simulink model "Auto_Coffee"  (R2017a)
settings: Solver=VariableStepAuto  StartTime=0.0  StopTime=25  RelTol=1e-3
undefined symbols (not defined in the file): sigbuilder_block
settings Model: Creator=Administrator  LastModifiedBy=Administrator
settings OptimizationCC: DefaultParameterBehavior=Inlined  UseDivisionForNetSlopeComputation=on  UseFloatMulNetSlope=on  InlineInvariantSignals=on  PassReuseOutputArgsAs=Individual arguments  ZeroExternalMemoryAtStartup=off  ZeroInternalMemoryAtStartup=off  NoFixptDivByZeroProtection=on  EfficientFloat2IntCast=on  LifeSpan=1
settings DebuggingCC: ParameterTunabilityLossMsg=error
settings HardwareCC: ProdBitPerPointer=32  ProdBitPerSizeT=32  ProdBitPerPtrDiffT=32  ProdLargestAtomicInteger=Long  ProdWordSize=32  ProdHWDeviceType=ARM Compatible->ARM 7
settings SFSimCC: MATLABDynamicMemAlloc=off
settings RTWCC: SystemTargetFile=ert.tlc  TemplateMakefile=ert_default_tmf  Description=Embedded Coder  GenerateReport=on  IncludeHyperlinkInReport=on  LaunchReport=on  GenerateTraceInfo=on  GenerateTraceReport=on  GenerateTraceReportSl=on  GenerateTraceReportSf=on  GenerateTraceReportEml=on  GenerateCodeMetricsReport=on
settings CodeAppCC: ForceParamTrailComments=on  IgnoreCustomStorageClasses=off  OperatorAnnotations=on  SimulinkDataObjDesc=on  SFDataObjDesc=on  MATLABFcnDesc=on  CustomSymbolStrGlobalVar=rt$N$M  CustomSymbolStrType=$N$M  CustomSymbolStrFcn=$N$M$F  CustomSymbolStrMacro=$N$M  InsertBlockDesc=on  MATLABSourceComments=on
settings ERTTargetCC: TargetLangStandard=C99 (ISO)  GenerateSampleERTMain=on  IncludeMdlTerminateFcn=off  CombineSignalStateStructs=on  SupportComplex=off  SupportContinuousTime=on  SupportNonInlinedSFcns=on  InlinedParameterPlacement=NonHierarchical  ERTCustomFileTemplate=example_file_process.tlc  ERTFilePackagingFormat=CompactWithDataFile

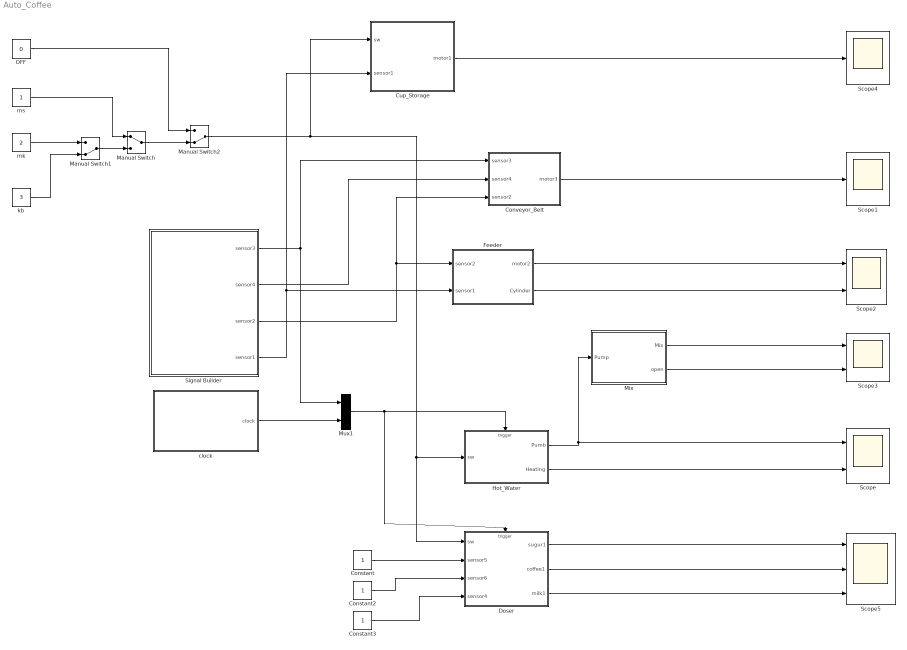
== system Auto_Coffee ==
  Constant : Constant
  Constant2 : Constant
  Constant3 : Constant
  Conveyor_Belt : Stateflow chart  TreatAsAtomicUnit=on
  Cup_Storage : Stateflow chart  TreatAsAtomicUnit=on
  Doser : Stateflow chart  TreatAsAtomicUnit=on
  Feeder : Stateflow chart  TreatAsAtomicUnit=on
  Hot_Water : Stateflow chart  TreatAsAtomicUnit=on
  Manual Switch : ManualSwitch
  Manual Switch1 : ManualSwitch  CurrentSetting=0
  Manual Switch2 : ManualSwitch  CurrentSetting=0
  Mix : Stateflow chart  TreatAsAtomicUnit=on
  Mux1 : Mux  Inputs=2
  OFF : Constant  Value=0
  Scope : Scope  NumInputPorts=2
  Scope1 : Scope
  Scope2 : Scope  NumInputPorts=2
  Scope3 : Scope  NumInputPorts=2
  Scope4 : Scope
  Scope5 : Scope  NumInputPorts=3
  Signal Builder : Subsystem  Tag=STV Subsys  LoadFcn=sigbuilder_block('load');  StartFcn=sigbuilder_block('start');  StopFcn=sigbuilder_block('stop');  ClipboardFcn=sigbuilder_block('clipboard');  mask(Sigbuilder block){tuvar=[0:10]}
      mask help: Simulink:masks:SigbuilderBlock_MD
      mask init:
      | if ~strcmp(get_param(bdroot(gcbh),'SimulationStatus'),'stopped') tuvar = sigbuilder_block('maskInit'); end
      settings: CopyFcn=sigbuilder_block('copy');  DeleteFcn=sigbuilder_block('delete');  ModelCloseFcn=sigbuilder_block('modelClose');  PreSaveFcn=sigbuilder_block('preSave');  PauseFcn=sigbuilder_block('pause');  ContinueFcn=sigbuilder_block('continue');  NameChangeFcn=sigbuilder_block('namechange');  OpenFcn=sigbuilder_block('open',[-90.75 166.5 572.25 408.75 ]);  CloseFcn=sigbuilder_block('close');
      mask Display: plot(0, 0, 100, 100,[2, 2, 32, 32, 2], [68, 8, 8, 68, 68],[32, 2], [38, 38], [32, 19, 2],[53, 60, 44], [32, 17, 17, 2],[16, 16, 31, 31]);txt = getActiveGroup(gcbh);text(2, 100, txt,'verticalAlignment', 'top');
  clock : Subsystem  Tag=STV Subsys  LoadFcn=sigbuilder_block('load');  StartFcn=sigbuilder_block('start');  StopFcn=sigbuilder_block('stop');  ClipboardFcn=sigbuilder_block('clipboard');  mask(Sigbuilder block){tuvar=[0:10]}
      mask help: Simulink:masks:SigbuilderBlock_MD
      mask init:
      | if ~strcmp(get_param(bdroot(gcbh),'SimulationStatus'),'stopped') tuvar = sigbuilder_block('maskInit'); end
      settings: CopyFcn=sigbuilder_block('copy');  DeleteFcn=sigbuilder_block('delete');  ModelCloseFcn=sigbuilder_block('modelClose');  PreSaveFcn=sigbuilder_block('preSave');  PauseFcn=sigbuilder_block('pause');  ContinueFcn=sigbuilder_block('continue');  NameChangeFcn=sigbuilder_block('namechange');  OpenFcn=sigbuilder_block('open',[517.5 155.25 550.5 358.5 ]);  CloseFcn=sigbuilder_block('close');
      mask Display: plot(0, 0, 100, 100,[2, 2, 32, 32, 2], [68, 8, 8, 68, 68],[32, 2], [38, 38], [32, 19, 2],[53, 60, 44], [32, 17, 17, 2],[16, 16, 31, 31]);txt = getActiveGroup(gcbh);text(2, 100, txt,'verticalAlignment', 'top');
  kb : Constant  Value=3
  mk : Constant  Value=2
  ms : Constant
  wires:
  Hot_Water/1(Pumb) -> Mix/1(Pump), Scope/1
  Hot_Water/2(Heating) -> Scope/2
  Signal Builder/1(sensor3) -> Conveyor_Belt/1(sensor3), Mux1/1
  Conveyor_Belt/1(motor3) -> Scope1/1
  Signal Builder/2(sensor4) -> Conveyor_Belt/2(sensor4)
  Signal Builder/3(sensor2) -> Conveyor_Belt/3(sensor2), Feeder/1(sensor2)
  Signal Builder/4(sensor1) -> Cup_Storage/2(sensor1), Feeder/2(sensor1)
  Feeder/1(motor2) -> Scope2/1
  Mix/1(Mix) -> Scope3/1
  Mix/2(open) -> Scope3/2
  Feeder/2(Cylinder) -> Scope2/2
  Cup_Storage/1(motor1) -> Scope4/1
  Constant/1 -> Doser/2(sensor5)
  Constant3/1 -> Doser/4(sensor4)
  Constant2/1 -> Doser/3(sensor6)
  clock/1(clock) -> Mux1/2
  Mux1/1 -> Hot_Water/Trigger, Doser/Trigger
  Manual Switch2/1 -> Hot_Water/1(sw), Doser/1(sw), Cup_Storage/1(sw)
  Manual Switch/1 -> Manual Switch2/2
  Manual Switch1/1 -> Manual Switch/2
  OFF/1 -> Manual Switch2/1
  ms/1 -> Manual Switch/1
  mk/1 -> Manual Switch1/1
  kb/1 -> Manual Switch1/2
  Doser/1(sugur1) -> Scope5/1
  Doser/2(coffee1) -> Scope5/2
  Doser/3(milk1) -> Scope5/3

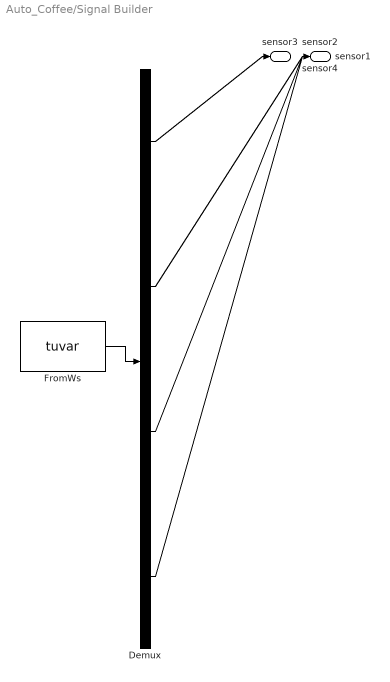
== system Auto_Coffee/Signal Builder ==
  Demux : Demux  Tag=STV Demux
  FromWs : FromWorkspace  Tag=STV FromWs  VariableName=tuvar  SampleTime=0
      SigBuilderData=|
      | common.afterFinalStr = 'Extrapolate'
      | common.sampleTime = 0
      | dataSet.timeRange = [0 25]
      | dataSet.name = 'Group 1'
      | sbobj.Groups.Name = 'Group 1'
      | sbobj.Groups.Signals(1).Name = 'sensor3'
      | sbobj.Groups.Signals(1).XData = [0 10 10 20 20 25]
      | sbobj.Groups.Signals(1).YData = [0 0 1 1 0 0]
      | sbobj.Groups.Signals(2).Name = 'sensor4'
      | sbobj.Groups.Signals(2).XData = [0 23 23 25]
      | sbobj.Groups.Signals(2).YData = [0 0 1 1]
      | sbobj.Groups.Signals(3).Name = 'sensor2'
      | sbobj.Groups.Signals(3).XData = [0 4 4 6 6 25]
      | sbobj.Groups.Signals(3).YData = [0 0 1 1 0 0]
      | sbobj.Groups.Signals(4).Name = 'sensor1'
      | sbobj.Groups.Signals(4).XData = [0 2 2 3 3 25]
      | sbobj.Groups.Signals(4).YData = [0 0 1 1 0 0]
      | sbobj.Groups.TimeRange = [0 25]
  sensor3 : Outport  Tag=STV Outport
  sensor4 : Outport  Tag=STV Outport  Port=2
  sensor2 : Outport  Tag=STV Outport  Port=3
  sensor1 : Outport  Tag=STV Outport  Port=4
  wires:
  FromWs/1 -> Demux/1
  Demux/1 -> sensor3/1
  Demux/2 -> sensor4/1
  Demux/3 -> sensor2/1
  Demux/4 -> sensor1/1

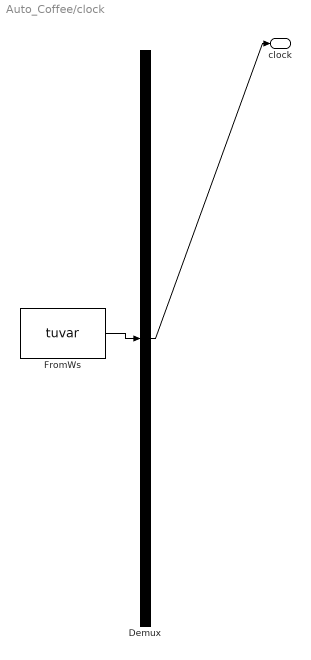
== system Auto_Coffee/clock ==
  Demux : Demux  Tag=STV Demux  Outputs=1
  FromWs : FromWorkspace  Tag=STV FromWs  VariableName=tuvar  SampleTime=0
      SigBuilderData=|
      | common.afterFinalStr = 'Extrapolate'
      | common.sampleTime = 0
      | dataSet.timeRange = [0 25]
      | dataSet.name = 'Group 1'
      | sbobj.Groups.Name = 'Group 1'
      | sbobj.Groups.Signals.Name = 'clock'
      | sbobj.Groups.Signals.XData = [0 0.25 0.25 0.5 0.5 0.75 0.75 1 1 1.25 1.25 1.5 1.5 1.75 1.75 2 2 2.25 2.25 2.5 2.5 2.75 2.75 3 3 3.25 3.25 3.5 3.5 3.75 3.75 4 4 4.25 4.25 4.5 4.5 4.75 4.75 5 5 5.25 5.25 5.5 5.5 5.75 5.75 6 6 6.25 6.25 6.5 6.5 6.75 6.75 7 7 7.25 7.25 7.5 7.5 7.75 7.75 8 8 8.25 8.25 8.5 8.5 8.75 8.75 9 9 9.25 9.25 9.5 9.5 9.75 9.75 10 10 10.25 10.25 10.5 10.5 10.75 10.75 11 11 11.25 11.25 11.5 11.5 11.75 11.75 12 12 12.25 12.25 12.5 12.5 12.75 12.75 13 13 13.25 13.25 13.5 13.5 13.75 13.75 14 14 14.25 14.25 14.5 14.5 14.75 14.75 15 15 15.25 15.25 15.5 15.5 15.75 15.75 16 16 16.25 16.25 16.5 16.5 16.75 16.75 17 17 17.25 17.25 17.5 17.5 17.75 17.75 18 18 18.25 18.25 18.5 18.5 18.75 18.75 19 19 19.25 19.25 19.5 19.5 19.75 19.75 20 20 20.25 20.25 20.5 20.5 20.75 20.75 21 21 21.25 21.25 21.5 21.5 21.75 21.75 22 22 22.25 22.25 22.5 22.5 22.75 22.75 23 23 23.25 23.25 23.5 23.5 23.75 23.75 24 24 24.25 24.25 24.5 24.5 24.75 24.75 25]
      | sbobj.Groups.Signals.YData = [2 2 0 0 2 2 0 0 2 2 0 0 2 2 0 0 2 2 0 0 2 2 0 0 2 2 0 0 2 2 0 0 2 2 0 0 2 2 0 0 2 2 0 0 2 2 0 0 2 2 0 0 2 2 0 0 2 2 0 0 2 2 0 0 2 2 0 0 2 2 0 0 2 2 0 0 2 2 0 0 2 2 0 0 2 2 0 0 2 2 0 0 2 2 0 0 2 2 0 0 2 2 0 0 2 2 0 0 2 2 0 0 2 2 0 0 2 2 0 0 2 2 0 0 2 2 0 0 2 2 0 0 2 2 0 0 2 2 0 0 2 2 0 0 2 2 0 0 2 2 0 0 2 2 0 0 2 2 0 0 2 2 0 0 2 2 0 0 2 2 0 0 2 2 0 0 2 2 0 0 2 2 0 0 2 2 0 0 2 2 0 0 2 2 0 0 2 2 0 0]
      | sbobj.Groups.TimeRange = [0 25]
  clock : Outport  Tag=STV Outport
  wires:
  FromWs/1 -> Demux/1
  Demux/1 -> clock/1

== stateflow chart Auto_Coffee/Conveyor_Belt ==
  state ON
    state motor_on
      en:motor3=1;
    state motor_off
      en:motor3=0;
    (default) -> motor_on
    motor_on -> motor_off : [sensor3==1]
    motor_off -> motor_on : after(10,sec)
  state OFF
    en:motor3=0;
  OFF -> ON : [sensor4==0&&sensor2==1]
  ON -> OFF : [sensor4==1&&sensor2==0]
  (default) -> OFF
  data: sensor3 input; sensor4 input; sensor2 input; motor3 output

== stateflow chart Auto_Coffee/Feeder ==
  state On
    en:motor2=1
  state OFF
    en:motor2=0
  state On1
    en:Cylinder=1
  state Off2
    en:Cylinder=0
  state OFF2
    en:motor2=0
  (default) -> OFF
  OFF -> On : [sensor1==1]
  On1 -> Off2 : after(1,sec)
  OFF2 -> On1 : after(1,sec)
  On -> OFF2 : [sensor2==1]
  data: motor2 output; sensor2 input; sensor1 input; Cylinder output

== stateflow chart Auto_Coffee/Hot_Water ==
  settings: executeAtInitialization=1
  state PowerOn
    state Pumb [parallel]
      settings: executionOrder=1
      state On
        en:Pumb=1;
      state Off
        en:Pumb=0;
      PowerOn.Pumb.On -> PowerOn.Pumb.Off : after(10,sec)
      PowerOn.Pumb.Off -> PowerOn.Pumb.On : sensor3
      (default) -> PowerOn.Pumb.Off
    state Heating [parallel]
      settings: executionOrder=2
      state On
        en:Heating=1;
      state Off
        en:Heating=0;
      PowerOn.Heating.On -> PowerOn.Heating.Off : after(10,sec)
      PowerOn.Heating.Off -> PowerOn.Heating.On : sensor3
      (default) -> PowerOn.Heating.Off
  state PowerOff
  PowerOff -> PowerOn : [sw~=0]
  PowerOn -> PowerOff : [sw==0]
  (default) -> PowerOff
  data: sw input; Pumb output; Heating output
  events: sensor3 input RISING_EDGE_EVENT; clock input RISING_EDGE_EVENT

== stateflow chart Auto_Coffee/Mix ==
  state off
    en:Mix=0;
    open=0;
  state wait
    en:Mix=0;
    open=0;
  state on
    en:Mix=0;
    open=1;
  state mix
    en:Mix=1;
  (default) -> off
  off -> wait : [Pump==1]
  on -> off : after(3,sec)
  wait -> mix : after(5,sec)
  mix -> on : after(2,sec)
  data: Pump input; Mix output; open output

== stateflow chart Auto_Coffee/Cup_Storage ==
  state on
    state motor_off
      en:motor1=0;
    state motor_on
      en:motor1=1;
      flag=1;
    motor_off -> motor_on : [sensor1==0&&flag==0]
    motor_on -> motor_off : after(1,sec)
    (default) -> motor_off
  state off
    en:motor1=0;
    flag=0;
  off -> on : [sw~=0]
  on -> off : [sw==0]
  (default) -> off
  data: sw input; motor1 output; sensor1 input; flag local

== stateflow chart Auto_Coffee/Doser ==
  settings: executeAtInitialization=1
  state on
    state coffee [parallel]
      settings: executionOrder=1
      state on
        en:coffee1=1
      state off
        en:coffee1=0
      on.coffee.on -> on.coffee.off : [sensor4==0||after(10,sec)]
      on.coffee.off -> on.coffee.on : [sw~=0&&sensor3&&sensor4==1]
      (default) -> on.coffee.off
    state milk [parallel]
      settings: executionOrder=2
      state on
        en:milk1=1
      state off
        en:milk1=0
      on.milk.on -> on.milk.off : [sensor5==0||after(10,sec)]
      on.milk.off -> on.milk.on : [(sw==2||sw==3)&&sensor3&&sensor5]
      (default) -> on.milk.off
    state sugur [parallel]
      settings: executionOrder=3
      state on
        en:sugur1=1
      state off
        en:sugur1=0
      on.sugur.on -> on.sugur.off : [sensor6==0||after(10,sec)]
      on.sugur.off -> on.sugur.on : [sw==3&&sensor3&&sensor6]
      (default) -> on.sugur.off
  state off
    en:coffee1=0;
    milk1=0;
    sugur1=0;
  on -> off : [sw==0]
  off -> on : [sw~=0]
  (default) -> off
  data: sw input; sensor5 input; sensor6 input; sensor4 input; sugur1 output; coffee1 output; milk1 output
  events: sensor3 input RISING_EDGE_EVENT; time input RISING_EDGE_EVENT
